simulink model "FederMitGewichtBeispiel"  (R2016b)
settings: Solver=FixedStepAuto  StartTime=0.0  StopTime=1000  FixedStep=0.01  RelTol=1e-3
settings Model: Creator=Thomas  LastModifiedBy=Thomas

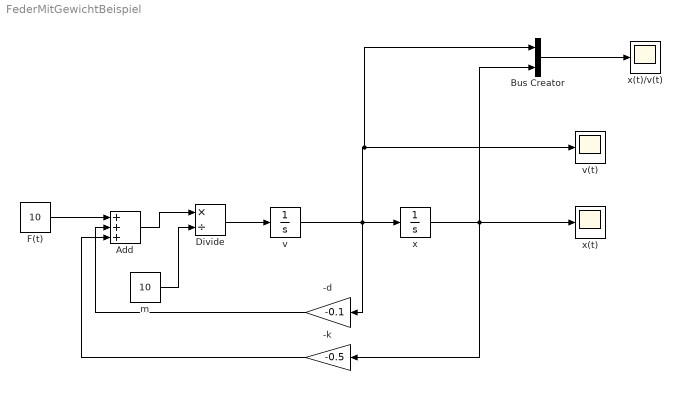
== system FederMitGewichtBeispiel ==
  "-d " : Gain  Gain=-0.1
  -k : Gain  Gain=-0.5
  Add : Sum  Inputs=+++
  Bus Creator : BusCreator  Inputs=2
  Divide : Product  Inputs=*/
  F(t) : Constant  Value=10
  m : Constant  Value=10
  "v " : Integrator
  v(t) : Scope
  x : Integrator
  x(t) : Scope
  x(t)/v(t) : Scope
  wires:
  F(t)/1 -> Add/1
  "v "/1 -> Bus Creator/1, v(t)/1, x/1, "-d "/1
  x/1 -> Bus Creator/2, x(t)/1, -k/1
  "-d "/1 -> Add/2
  -k/1 -> Add/3
  Divide/1 -> "v "/1
  m/1 -> Divide/2
  Add/1 -> Divide/1
  Bus Creator/1 -> x(t)/v(t)/1
